simulink model "Modelo_global_NL_con_LC_NL_backup"  (R2023a)
settings: Solver=VariableStepAuto  StartTime=0.0  StopTime=10.0  RelTol=1e-3
model workspace: external: MAT-File C:\Users\tobip\Documents\Ayme\Matlab\datos.mat (data not in the file)
values from neighbouring files (symbols this model uses):
  k_l = m*g*l_cm + m_l*g*l_l    (= 9.80665)    [variables.m]
  r = 120    [variables.m]
undefined symbols (not defined in the file or in its folder): alpha_Cu, b_eq, Cts, J_eq, lambda, Ld, Lls, Lq, Pp, Rts, Ts_ref
settings Model: Creator=Renzo  LastModifiedBy=tobip
settings DataIOCC: ExternalInput=vqs,T_amb,Tp  LoadExternalInput=on

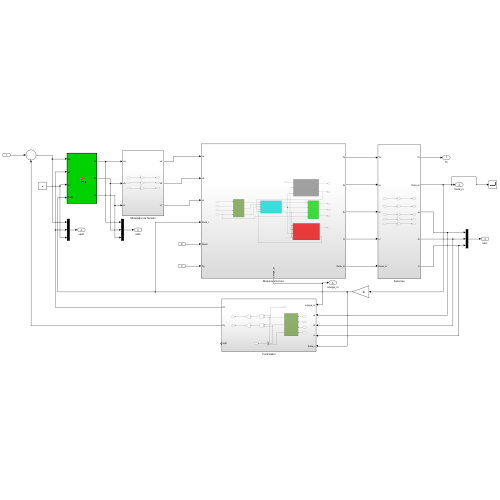
[thumbnail: Simulink's stored preview of the top-level diagram]
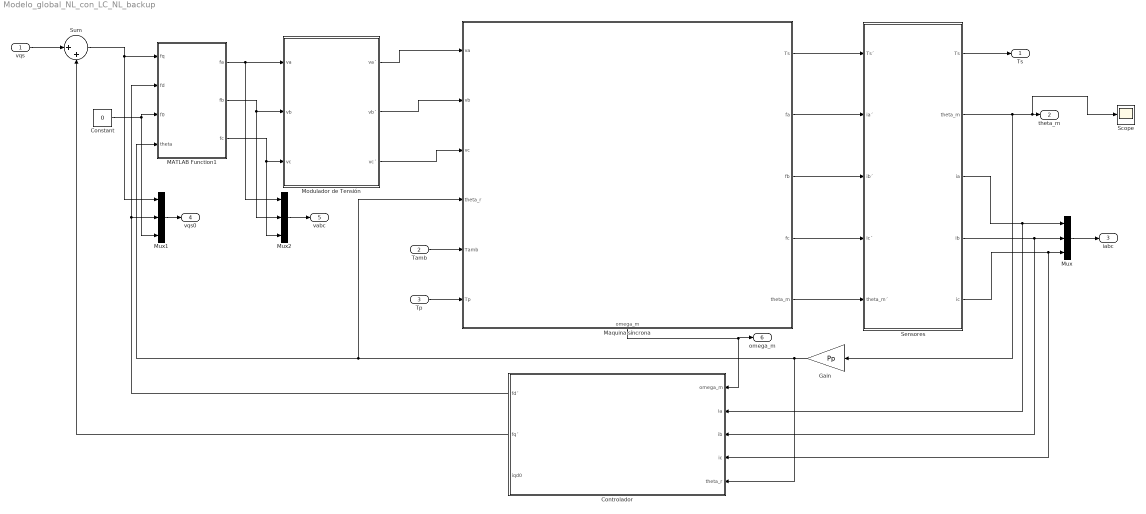
== system Modelo_global_NL_con_LC_NL_backup ==
  vqs : Inport
  Tamb : Inport  Port=2
  Tp : Inport  Port=3
  Constant : Constant  Value=0
  Controlador : Subsystem
  Gain : Gain  Gain=Pp
  MATLAB Function1 : MATLAB Function  TreatAsAtomicUnit=on
  Maquina síncrona : Subsystem
      settings: PortSchema="{\"entries\":[{\"content\":{\"sides\":[{\"content\":{\"connectorIds\":[\"In1\",\"In2\",\"In3\",\"In4\",\"In5\",\"In6\"]},\"type\":\"ConnectorPlacement.EquallySpacedRectSide\",\"uuid\":\"548fbf6f-bb54-461c-a3ca-ae13566b19bb\"},{\"content\":{\"connectorIds\":[\"Out1\",\"Out2\",\"Out3\",\"Out4\",\"Out5\"],\"side\":\"RIGHT\"},\"type\":\"ConnectorPlacement.EquallySpacedRectSide\",\"uuid\":\"c9a1420a-e64d-4e02-ad2b-140f5c663a2c\"},{\"content\":{\"side\":\"TOP\"},\"type\":\"ConnectorPlacement.EquallySpacedRectSide\",\"uuid\":\"df4aae34-4e90-4058-9a3e-cb814e1189cf\"},{\"content\":{\"connectorIds\":[\"Out6\"],\"side\":\"BOTTOM\"},\"type\":\"ConnectorPlacement.EquallySpacedRectSide\",\"uuid\":\"ac35aa20-eac6-4ff0-8145-8d4a0e731d5f\"}]},\"type\":\"ConnectorPlacement.EquallySpacedConnector\",\"uuid\":\"8e0529f1-5fe4-4179-9319-aba0984f7167\"}],\"packageUris\":[\"http://schema.mathworks.com/mf0/Connector/R2020b\"],\"version\":\"1.0\"}"
  Modulador de Tensión : Subsystem
  Mux : Mux  Inputs=3
  Mux1 : Mux  Inputs=3
  Mux2 : Mux  Inputs=3
  Scope : Scope
  Sensores : Subsystem
  Sum : Sum  Inputs=|++
  Ts : Outport
  theta_m : Outport  Port=2
  iabc : Outport  Port=3
  vqs0 : Outport  Port=4
  vabc : Outport  Port=5
  omega_m : Outport  Port=6
  wires:
  Modulador de Tensión/1(va´) -> Maquina síncrona/1(va)
  Modulador de Tensión/2(vb´) -> Maquina síncrona/2(vb)
  Modulador de Tensión/3(vc´) -> Maquina síncrona/3(vc)
  MATLAB Function1/1(fa) -> Modulador de Tensión/1(va), Mux2/1
  MATLAB Function1/2(fb) -> Modulador de Tensión/2(vb), Mux2/2
  MATLAB Function1/3(fc) -> Modulador de Tensión/3(vc), Mux2/3
  Maquina síncrona/1(Ts) -> Sensores/1(Ts´)
  Maquina síncrona/2(fa) -> Sensores/2(ia´)
  Maquina síncrona/3(fb) -> Sensores/3(ib´)
  Maquina síncrona/4(fc) -> Sensores/4(ic´)
  Maquina síncrona/5(theta_m) -> Sensores/5(theta_m´)
  Sensores/1(Ts) -> Ts/1
  Sensores/2(theta_m) -> Scope/1, theta_m/1, Gain/1
  Sensores/3(ia) -> Controlador/2(ia), Mux/1
  Sensores/4(ib) -> Controlador/3(ib), Mux/2
  Sensores/5(ic) -> Mux/3, Controlador/4(ic)
  Mux/1 -> iabc/1
  Controlador/2(fq´) -> Sum/2
  Sum/1 -> Mux1/1, MATLAB Function1/1(fq)
  vqs/1 -> Sum/1
  Constant/1 -> MATLAB Function1/3(f0), Mux1/3
  Controlador/1(fd´) -> MATLAB Function1/2(fd), Mux1/2
  Mux1/1 -> vqs0/1
  Mux2/1 -> vabc/1
  Gain/1 -> Controlador/5(theta_r), MATLAB Function1/4(theta), Maquina síncrona/4(theta_r)
  Tp/1 -> Maquina síncrona/6(Tp)
  Tamb/1 -> Maquina síncrona/5(Tamb)
  Maquina síncrona/6(omega_m) -> omega_m/1, Controlador/1(omega_m)

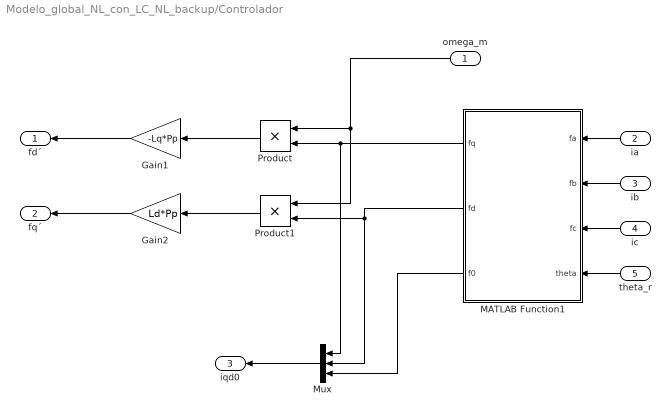
== system Modelo_global_NL_con_LC_NL_backup/Controlador ==
  omega_m : Inport
  ia : Inport  Port=2
  ib : Inport  Port=3
  ic : Inport  Port=4
  theta_r : Inport  Port=5
  Gain1 : Gain  Gain=-Lq*Pp
  Gain2 : Gain  Gain=Ld*Pp
  MATLAB Function1 : MATLAB Function  TreatAsAtomicUnit=on
  Mux : Mux  Inputs=3
  Product : Product
  Product1 : Product
  fd´ : Outport
  fq´ : Outport  Port=2
  iqd0 : Outport  Port=3
  wires:
  ia/1 -> MATLAB Function1/1(fa)
  ib/1 -> MATLAB Function1/2(fb)
  ic/1 -> MATLAB Function1/3(fc)
  theta_r/1 -> MATLAB Function1/4(theta)
  omega_m/1 -> Product/1, Product1/1
  MATLAB Function1/1(fq) -> Mux/1, Product/2
  MATLAB Function1/2(fd) -> Product1/2, Mux/2
  MATLAB Function1/3(f0) -> Mux/3
  Product1/1 -> Gain2/1
  Product/1 -> Gain1/1
  Mux/1 -> iqd0/1
  Gain1/1 -> fd´/1
  Gain2/1 -> fq´/1

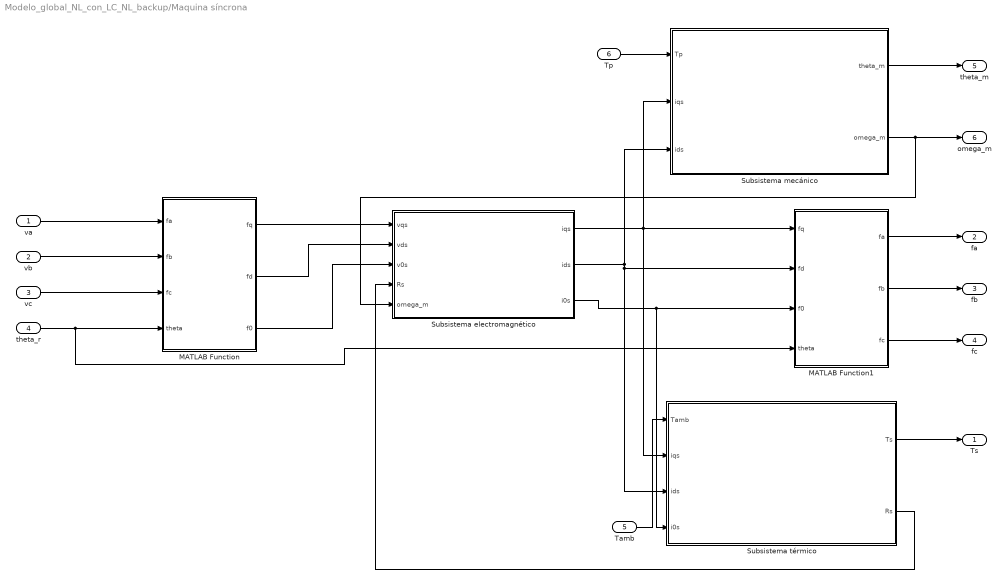
== system Modelo_global_NL_con_LC_NL_backup/Maquina síncrona ==
  va : Inport
  vb : Inport  Port=2
  vc : Inport  Port=3
  theta_r : Inport  Port=4
  Tamb : Inport  Port=5
  Tp : Inport  Port=6
  MATLAB Function : MATLAB Function  TreatAsAtomicUnit=on
  MATLAB Function1 : MATLAB Function  TreatAsAtomicUnit=on
  Subsistema electromagnético : Subsystem
  Subsistema mecánico : Subsystem
  Subsistema térmico : Subsystem
  Ts : Outport
  fa : Outport  Port=2
  fb : Outport  Port=3
  fc : Outport  Port=4
  theta_m : Outport  Port=5
  omega_m : Outport  Port=6
  wires:
  theta_r/1 -> MATLAB Function/4(theta), MATLAB Function1/4(theta)
  Subsistema mecánico/2(omega_m) -> omega_m/1, Subsistema electromagnético/5(omega_m)
  va/1 -> MATLAB Function/1(fa)
  vc/1 -> MATLAB Function/3(fc)
  Subsistema electromagnético/2(ids) -> Subsistema térmico/3(ids), MATLAB Function1/2(fd), Subsistema mecánico/3(ids)
  MATLAB Function/3(f0) -> Subsistema electromagnético/3(v0s)
  MATLAB Function/2(fd) -> Subsistema electromagnético/2(vds)
  Tp/1 -> Subsistema mecánico/1(Tp)
  Tamb/1 -> Subsistema térmico/1(Tamb)
  MATLAB Function/1(fq) -> Subsistema electromagnético/1(vqs)
  Subsistema electromagnético/3(i0s) -> MATLAB Function1/3(f0), Subsistema térmico/4(i0s)
  Subsistema electromagnético/1(iqs) -> MATLAB Function1/1(fq), Subsistema térmico/2(iqs), Subsistema mecánico/2(iqs)
  MATLAB Function1/2(fb) -> fb/1
  MATLAB Function1/1(fa) -> fa/1
  MATLAB Function1/3(fc) -> fc/1
  vb/1 -> MATLAB Function/2(fb)
  Subsistema térmico/2(Rs) -> Subsistema electromagnético/4(Rs)
  Subsistema térmico/1(Ts) -> Ts/1
  Subsistema mecánico/1(theta_m) -> theta_m/1

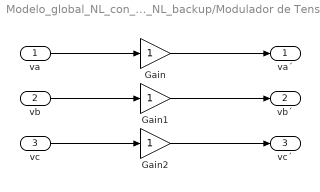
== system Modelo_global_NL_con_LC_NL_backup/Modulador de Tensión ==
  va : Inport
  vb : Inport  Port=2
  vc : Inport  Port=3
  Gain : Gain
  Gain1 : Gain
  Gain2 : Gain
  va´ : Outport
  vb´ : Outport  Port=2
  vc´ : Outport  Port=3
  wires:
  va/1 -> Gain/1
  Gain/1 -> va´/1
  vb/1 -> Gain1/1
  Gain1/1 -> vb´/1
  vc/1 -> Gain2/1
  Gain2/1 -> vc´/1

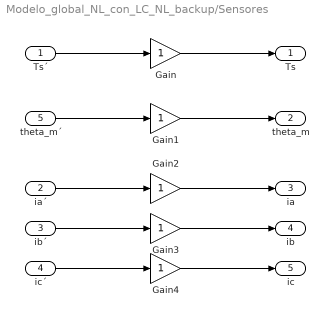
== system Modelo_global_NL_con_LC_NL_backup/Sensores ==
  Ts´ : Inport
  ia´ : Inport  Port=2
  ib´ : Inport  Port=3
  ic´ : Inport  Port=4
  theta_m´ : Inport  Port=5
  Gain{,1..4} (5 alike) : Gain
  Ts : Outport
  theta_m : Outport  Port=2
  ia : Outport  Port=3
  ib : Outport  Port=4
  ic : Outport  Port=5
  wires:
  Ts´/1 -> Gain/1
  Gain/1 -> Ts/1
  theta_m´/1 -> Gain1/1
  Gain1/1 -> theta_m/1
  ia´/1 -> Gain2/1
  Gain2/1 -> ia/1
  ib´/1 -> Gain3/1
  Gain3/1 -> ib/1
  ic´/1 -> Gain4/1
  Gain4/1 -> ic/1

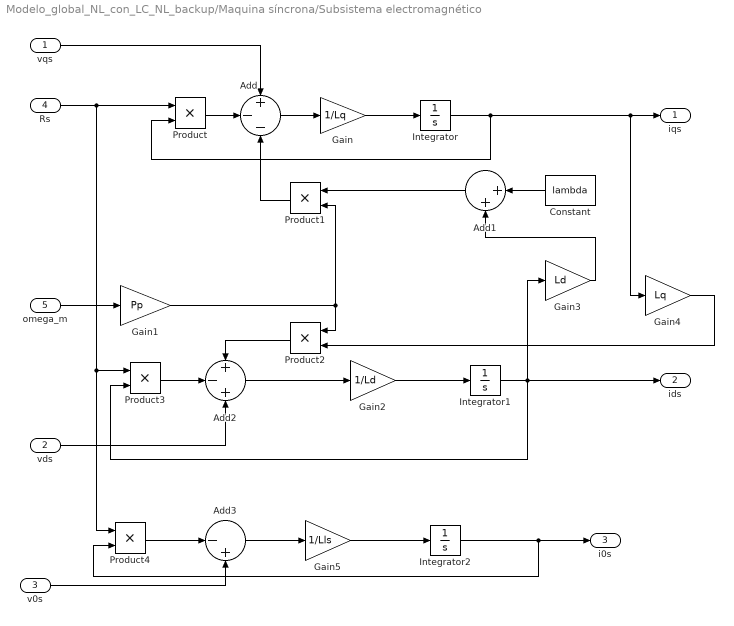
== system Modelo_global_NL_con_LC_NL_backup/Maquina síncrona/Subsistema electromagnético ==
  vqs : Inport
  vds : Inport  Port=2
  v0s : Inport  Port=3
  Rs : Inport  Port=4
  omega_m : Inport  Port=5
  Add : Sum  Inputs=+--
  Add1 : Sum  Inputs=|++
  Add2 : Sum  Inputs=+-+
  Add3 : Sum  Inputs=|-+
  Constant : Constant  Value=lambda
  Gain : Gain  Gain=1/Lq
  Gain1 : Gain  Gain=Pp
  Gain2 : Gain  Gain=1/Ld
  Gain3 : Gain  Gain=Ld
  Gain4 : Gain  Gain=Lq
  Gain5 : Gain  Gain=1/Lls
  Integrator : Integrator
  Integrator1 : Integrator
  Integrator2 : Integrator
  Product{,1..4} (5 alike) : Product
  iqs : Outport
  ids : Outport  Port=2
  i0s : Outport  Port=3
  wires:
  vqs/1 -> Add/1
  Gain/1 -> Integrator/1
  Add/1 -> Gain/1
  Integrator/1 -> Product/2, Gain4/1, iqs/1
  Product/1 -> Add/2
  Rs/1 -> Product/1, Product4/1, Product3/1
  Constant/1 -> Add1/1
  Add1/1 -> Product1/1
  Gain1/1 -> Product2/1, Product1/2
  Product1/1 -> Add/3
  omega_m/1 -> Gain1/1
  Product2/1 -> Add2/1
  vds/1 -> Add2/3
  Product3/1 -> Add2/2
  Add2/1 -> Gain2/1
  Gain2/1 -> Integrator1/1
  Integrator1/1 -> Gain3/1, ids/1, Product3/2
  Gain4/1 -> Product2/2
  Gain3/1 -> Add1/2
  v0s/1 -> Add3/2
  Product4/1 -> Add3/1
  Add3/1 -> Gain5/1
  Gain5/1 -> Integrator2/1
  Integrator2/1 -> Product4/2, i0s/1

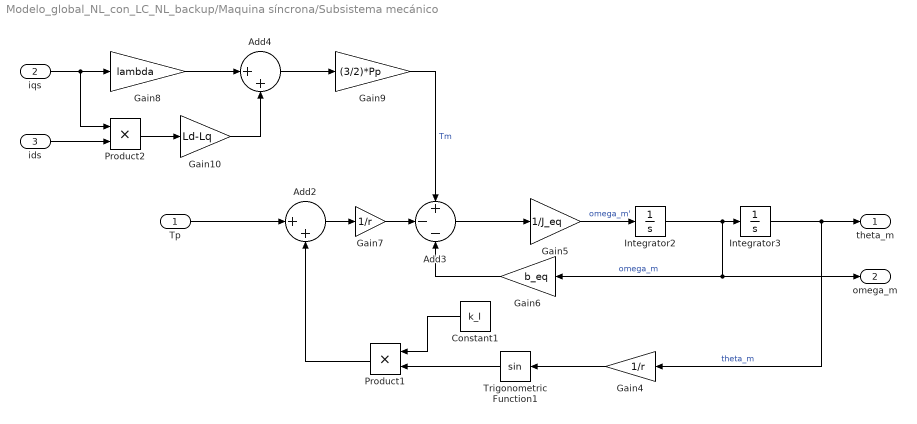
== system Modelo_global_NL_con_LC_NL_backup/Maquina síncrona/Subsistema mecánico ==
  Tp : Inport
  iqs : Inport  Port=2
  ids : Inport  Port=3
  Add2 : Sum  Inputs=|++
  Add3 : Sum  Inputs=+--
  Add4 : Sum  Inputs=|++
  Constant1 : Constant  Value=k_l
  Gain10 : Gain  Gain=Ld-Lq
  Gain4 : Gain  Gain=1/r
  Gain5 : Gain  Gain=1/J_eq
  Gain6 : Gain  Gain=b_eq
  Gain7 : Gain  Gain=1/r
  Gain8 : Gain  Gain=lambda
  Gain9 : Gain  Gain=(3/2)*Pp
  Integrator2 : Integrator
  Integrator3 : Integrator
  Product1 : Product
  Product2 : Product
  Trigonometric Function1 : Trigonometry
  theta_m : Outport
  omega_m : Outport  Port=2
  wires:
  Add2/1 -> Gain7/1
  Integrator2/1 -> omega_m/1, Gain6/1, Integrator3/1  "omega_m"
  Gain6/1 -> Add3/3
  Gain4/1 -> Trigonometric Function1/1
  Integrator3/1 -> theta_m/1, Gain4/1  "theta_m"
  iqs/1 -> Product2/1, Gain8/1
  Product1/1 -> Add2/2
  Add3/1 -> Gain5/1
  Gain5/1 -> Integrator2/1  "omega_m'"
  Constant1/1 -> Product1/1
  Tp/1 -> Add2/1
  Trigonometric Function1/1 -> Product1/2
  Gain8/1 -> Add4/1
  Gain7/1 -> Add3/2
  Add4/1 -> Gain9/1
  Gain9/1 -> Add3/1  "Tm"
  Product2/1 -> Gain10/1
  Gain10/1 -> Add4/2
  ids/1 -> Product2/2

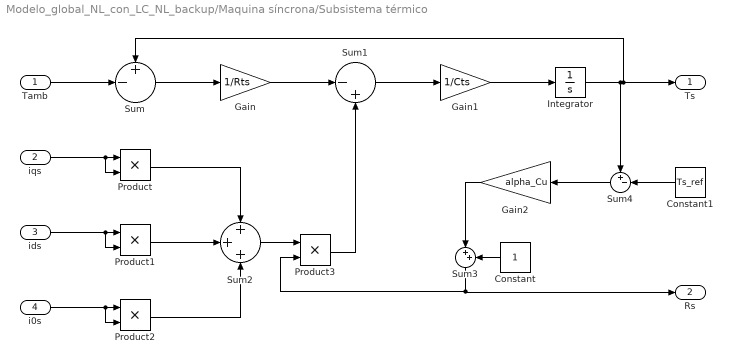
== system Modelo_global_NL_con_LC_NL_backup/Maquina síncrona/Subsistema térmico ==
  Tamb : Inport
  iqs : Inport  Port=2
  ids : Inport  Port=3
  i0s : Inport  Port=4
  Constant : Constant
  Constant1 : Constant  Value=Ts_ref
  Gain : Gain  Gain=1/Rts
  Gain1 : Gain  Gain=1/Cts
  Gain2 : Gain  Gain=alpha_Cu
  Integrator : Integrator
  Product{,1..3} (4 alike) : Product
  Sum : Sum  Inputs=+-|
  Sum1 : Sum  Inputs=|-+
  Sum2 : Sum  Inputs=+++
  Sum3 : Sum  Inputs=|++
  Sum4 : Sum  Inputs=+-|
  Ts : Outport
  Rs : Outport  Port=2
  wires:
  Tamb/1 -> Sum/2
  Gain/1 -> Sum1/1
  Sum/1 -> Gain/1
  Sum1/1 -> Gain1/1
  Gain1/1 -> Integrator/1
  Integrator/1 -> Ts/1, Sum/1, Sum4/1
  iqs/1 -> Product/2, Product/1
  ids/1 -> Product1/2, Product1/1
  i0s/1 -> Product2/2, Product2/1
  Product1/1 -> Sum2/2
  Product/1 -> Sum2/1
  Product2/1 -> Sum2/3
  Sum2/1 -> Product3/1
  Product3/1 -> Sum1/2
  Constant/1 -> Sum3/2
  Gain2/1 -> Sum3/1
  Constant1/1 -> Sum4/2
  Sum4/1 -> Gain2/1
  Sum3/1 -> Product3/2, Rs/1

== matlab function Modelo_global_NL_con_LC_NL_backup/Maquina síncrona/MATLAB Function1 ==
  data: fq input; fa output; fd input; f0 input; theta input; fb output; fc output
function [fa,fb,fc] = TI_Park(fq,fd,f0,theta)

f = (2/3)*[     cos(theta)              sin(theta)         1;
           cos(theta - (2*pi)/3)   sin(theta - (2*pi)/3)   1;
           cos(theta + (2*pi)/3)   sin(theta + (2*pi)/3)   1];

resultados = f*[fq;fd;f0];
fa = resultados(0);
fb = resultados(1);
fc = resultados(2);

== matlab function Modelo_global_NL_con_LC_NL_backup/Maquina síncrona/MATLAB Function ==
  data: fa input; fq output; fb input; fc input; theta input; fd output; f0 output
function [fq,fd,f0] = TD_Park(fa,fb,fc,theta)

f = (2/3)*[cos(theta)  cos(theta - (2*pi)/3)   cos(theta + (2*pi)/3);
           sin(theta)  sin(theta - (2*pi)/3)   sin(theta + (2*pi)/3);
              1/2              1/2                     1/2         ];

resultados = f*[fa;fb;fc];
fq = resultados(0);
fd = resultados(1);
f0 = resultados(2);

== matlab function Modelo_global_NL_con_LC_NL_backup/MATLAB Function1 ==
  data: fq input; fa output; fd input; f0 input; theta input; fb output; fc output
function [fa,fb,fc] = TI_Park(fq,fd,f0,theta)

f = (2/3)*[     cos(theta)              sin(theta)         1;
           cos(theta - (2*pi)/3)   sin(theta - (2*pi)/3)   1;
           cos(theta + (2*pi)/3)   sin(theta + (2*pi)/3)   1];

resultados = f*[fq;fd;f0];
fa = resultados(0);
fb = resultados(1);
fc = resultados(2);

== matlab function Modelo_global_NL_con_LC_NL_backup/Controlador/MATLAB Function1 ==
  data: fa input; fq output; fb input; fc input; theta input; fd output; f0 output
function [fq,fd,f0] = TD_Park(fa,fb,fc,theta)

f = (2/3)*[cos(theta)  cos(theta - (2*pi)/3)   cos(theta + (2*pi)/3);
           sin(theta)  sin(theta - (2*pi)/3)   sin(theta + (2*pi)/3);
              1/2              1/2                     1/2         ];

resultados = f*[fa;fb;fc];
fq = resultados(0);
fd = resultados(1);
f0 = resultados(2);
